simulink model "ITMBS_LEGO_Circle"  (R2023a)
settings: Solver=FixedStepDiscrete  StartTime=0.0  StopTime=30  FixedStep=0.05  RelTol=1e-3
undefined symbols (not defined in the file): sigbuilder_block
libraries: legoev3lib x3
settings Model: Creator=3w07  LastModifiedBy=manis
settings OptimizationCC: ReuseModelBlockBuffer=off

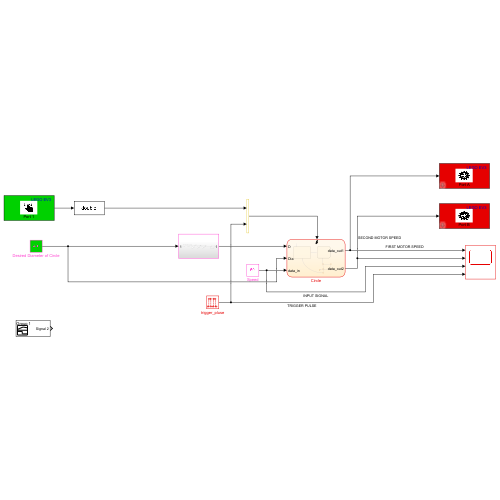
[thumbnail: Simulink's stored preview of the top-level diagram]
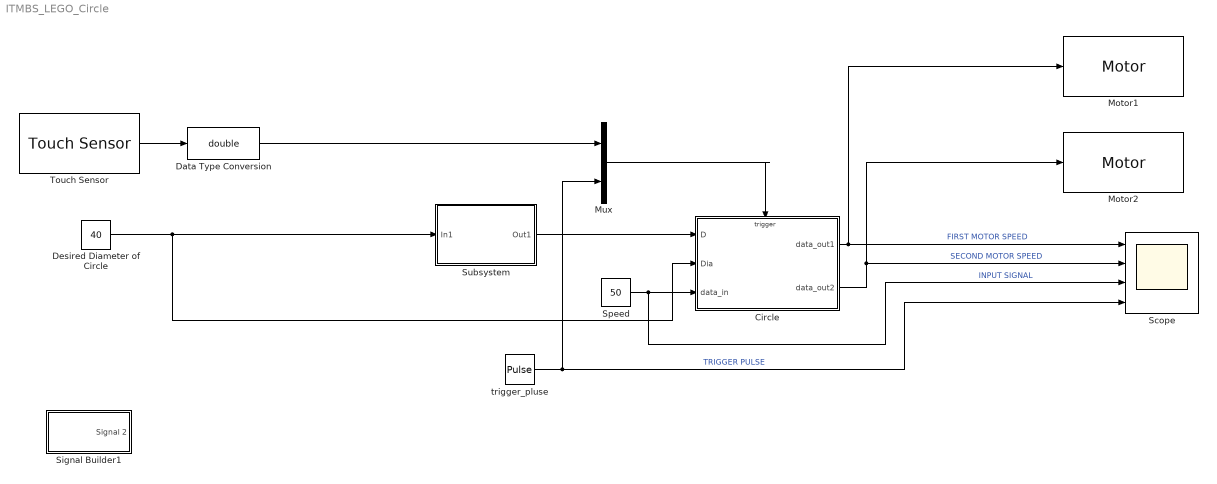
== system ITMBS_LEGO_Circle ==
  Circle : Stateflow chart  TreatAsAtomicUnit=on
  Data Type Conversion : DataTypeConversion  OutDataTypeStr=double  SaturateOnIntegerOverflow=off  RndMeth=Floor
  Desired Diameter of Circle : Constant  Value=40
  Motor1 : legoev3lib/Motor  sportNumber=A  sstopAction=Brake
  Motor2 : legoev3lib/Motor  sportNumber=B  sstopAction=Brake
  Mux : Mux  Inputs=2
  Scope : Scope  NumInputPorts=4
  Signal Builder1 : Subsystem  Tag=STV Subsys  LoadFcn=sigbuilder_block('load');  StartFcn=sigbuilder_block('start');  StopFcn=sigbuilder_block('stop');  ClipboardFcn=sigbuilder_block('clipboard');  mask(Sigbuilder block){tuvar=[0:10]}
      mask help: Simulink:masks:SigbuilderBlock_MD
      mask init:
      | if ~strcmp(get_param(bdroot(gcbh),'SimulationStatus'),'stopped') tuvar = sigbuilder_block('maskInit'); end
      settings: CopyFcn=sigbuilder_block('copy');  DeleteFcn=sigbuilder_block('delete');  ModelCloseFcn=sigbuilder_block('modelClose');  PreSaveFcn=sigbuilder_block('preSave');  PauseFcn=sigbuilder_block('pause');  ContinueFcn=sigbuilder_block('continue');  NameChangeFcn=sigbuilder_block('namechange');  OpenFcn=sigbuilder_block('open',[5.4 36 1141.2 516.6 ]);  CloseFcn=sigbuilder_block('close');
      mask Display: plot(0, 0, 100, 100,[2, 2, 32, 32, 2], [68, 8, 8, 68, 68],[32, 2], [38, 38], [32, 19, 2],[53, 60, 44], [32, 17, 17, 2],[16, 16, 31, 31]);txt = getActiveGroup(gcbh);text(2, 100, txt,'verticalAlignment', 'top');
  Speed : Constant  Value=50
  Subsystem : Subsystem
  Touch Sensor : legoev3lib/Touch Sensor  portNumber=1  sampleTime=0.1
  trigger_pluse : DiscretePulseGenerator  Period=10  PulseWidth=2  SampleTime=0.05
  wires:
  trigger_pluse/1 -> Mux/2, Scope/4  "TRIGGER PULSE"
  Speed/1 -> Scope/3, Circle/3(data_in)  "INPUT SIGNAL"
  Circle/1(data_out1) -> Motor1/1, Scope/1  "FIRST MOTOR SPEED"
  Circle/2(data_out2) -> Scope/2, Motor2/1  "SECOND MOTOR SPEED"
  Mux/1 -> Circle/Trigger
  Desired Diameter of Circle/1 -> Subsystem/1(In1), Circle/2(Dia)
  Subsystem/1(Out1) -> Circle/1(D)
  Touch Sensor/1 -> Data Type Conversion/1
  Data Type Conversion/1 -> Mux/1

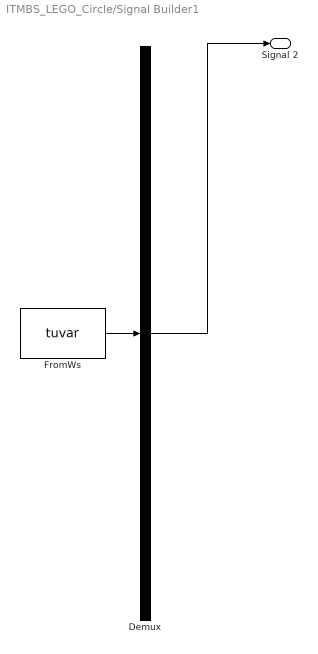
== system ITMBS_LEGO_Circle/Signal Builder1 ==
  Demux : Demux  Tag=STV Demux  Outputs=1
      settings: DisplayOption=none
  FromWs : FromWorkspace  Tag=STV FromWs  VariableName=tuvar
      SigBuilderData=|
      | common.afterFinalStr = 'Extrapolate'
      | common.sampleTime = 0
      | dataSet.timeRange = [0 20]
      | dataSet.name = 'Group 1'
      | sbobj.Groups.Name = 'Group 1'
      | sbobj.Groups.Signals.Name = 'Signal 2'
      | sbobj.Groups.Signals.XData = [0 4.19 4.19 4.28 4.28 6.036 6.301 6.301 6.401 6.401 6.499 6.499 6.601 6.601 20]
      | sbobj.Groups.Signals.YData = [0 0 1 1 0 0 0 0.995 0.995 0 0 0.995 0.995 0 0]
      | sbobj.Groups.TimeRange = [0 20]
  Signal 2 : Outport  Tag=STV Outport
  wires:
  FromWs/1 -> Demux/1
  Demux/1 -> Signal 2/1

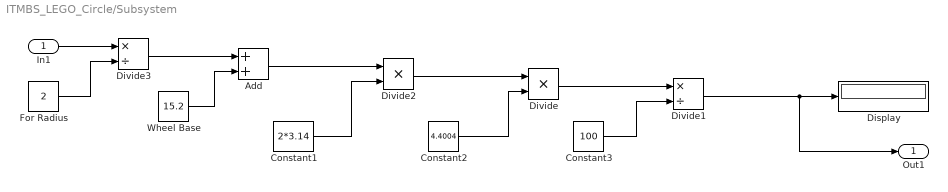
== system ITMBS_LEGO_Circle/Subsystem ==
  In1 : Inport
  Add : Sum
  Constant1 : Constant  Value=2*3.14
  Constant2 : Constant  Value=4.4004
  Constant3 : Constant  Value=100
  Display : Display
  Divide : Product  Inputs=**
  Divide1 : Product  Inputs=*/
  Divide2 : Product  Inputs=**
  Divide3 : Product  Inputs=*/
  For Radius : Constant  Value=2
  Wheel Base : Constant  Value=15.2
  Out1 : Outport
  wires:
  Divide3/1 -> Add/1
  For Radius/1 -> Divide3/2
  In1/1 -> Divide3/1
  Constant2/1 -> Divide/2
  Constant1/1 -> Divide2/2
  Divide2/1 -> Divide/1
  Wheel Base/1 -> Add/2
  Add/1 -> Divide2/1
  Divide/1 -> Divide1/1
  Constant3/1 -> Divide1/2
  Divide1/1 -> Out1/1, Display/1

== stateflow chart ITMBS_LEGO_Circle/Circle ==
  state LEGO_Run
    data_out1=data_in
    data_out2=(data_out1*(Dia-15.2))/(Dia+15.2)
  state LEGO_Stop
    data_out1=0;
    data_out2=0;
    entry:
    counter=0;
  (default) -> LEGO_Run
  LEGO_Run -> LEGO_Stop : [pb_event || after(D,sec)]
  LEGO_Stop -> (junction 26) : %pb_event
  (junction 45) -> LEGO_Run : [counter==2]
  (junction 26) -> (junction 28) [order 1] : [pb_event]
  (junction 26) -> (junction 42) [order 2]
  (junction 28) -> (junction 29) : {counter=counter+1}
  (junction 29) -> (junction 42)
  (junction 42) -> (junction 49) [order 2]
  (junction 42) -> (junction 45) [order 1]
  data: D input; Dia input; data_in input; data_out1 output; counter local; data_out2 output
  events: pb_event input RISING_EDGE_EVENT; event input RISING_EDGE_EVENT
